simulink model "Dynamic_vibration_absorber"  (R2020b)
settings: Solver=VariableStepAuto  StartTime=0.0  StopTime=10  RelTol=1e-3
PreLoadFcn:
  | %Problem 1 - Dynamic vibration absorber
  | %Values for the model
  | 
  | b=50
  | k1=50
  | k12=50
  | m1=100
  | m2=100
model workspace (MAT data in the model file):
  b = 50
  k1 = 50
  k12 = 50
  m1 = 100
  m2 = 100
settings Model: Creator=user  LastModifiedBy=user

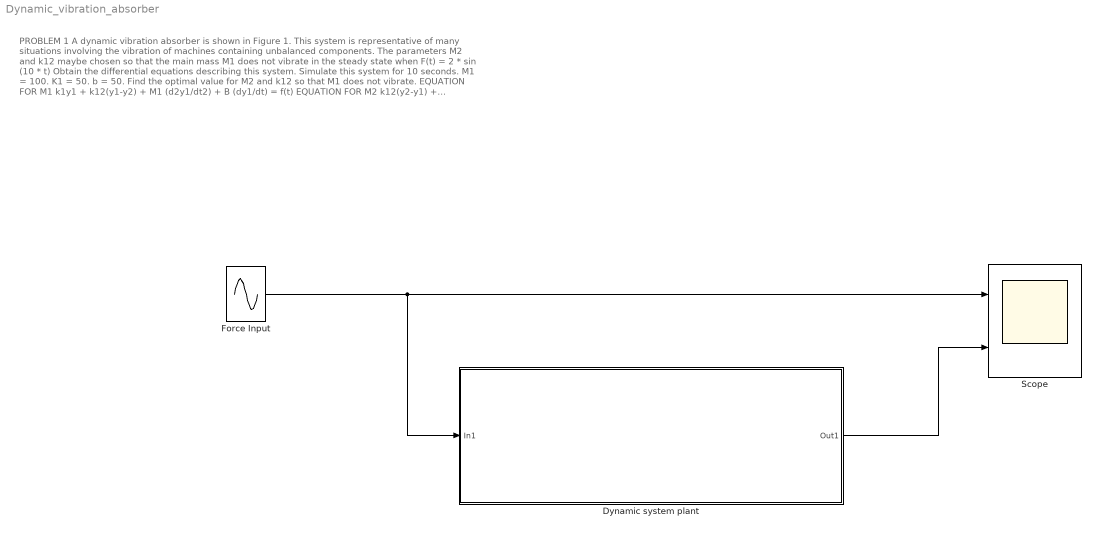
== system Dynamic_vibration_absorber ==
  note: PROBLEM 1
      |
      | A dynamic vibration absorber is shown in Figure 1. This system is representative of many situations involving the vibration of machines containing unbalanced components. The parameters M2 and k12 maybe chosen so that the main mass M1 does not vibrate in the steady state when F(t) = 2 * sin (10 * t) Obtain the differential equations describing this system. Simulate this system for 10 seconds. M1 = 100. K1 = 50. b = 50. Find the optimal value for M2 and k12 so that M1 does not vibrate.
      |
      | EQUATION FOR M1
      | k1y1 + k12(y1-y2) + M1 (d2y1/dt2) + B (dy1/dt) = f(t)
      |
      | EQUATION FOR M2
      | k12(y2-y1) + M2(d2y2/dt2) = 0
  "Dynamic system plant " : Subsystem  mask{m2=4, k12=25}
      mask prompts: m2 "Mass(m2)"; k12 "Spring Constant(k12)"
      mask Display: image('C:\Users\user\Downloads\Screenshot_20210307-220826.jpg'); % Use "Edit Image" on toolstrip to change.
  Force Input : Sin  Amplitude=2  Frequency=10  SampleTime=0
  "Scope " : Scope  NumInputPorts=2
  wires:
  Force Input/1 -> "Dynamic system plant "/1(In1), "Scope "/1
  "Dynamic system plant "/1(Out1) -> "Scope "/2

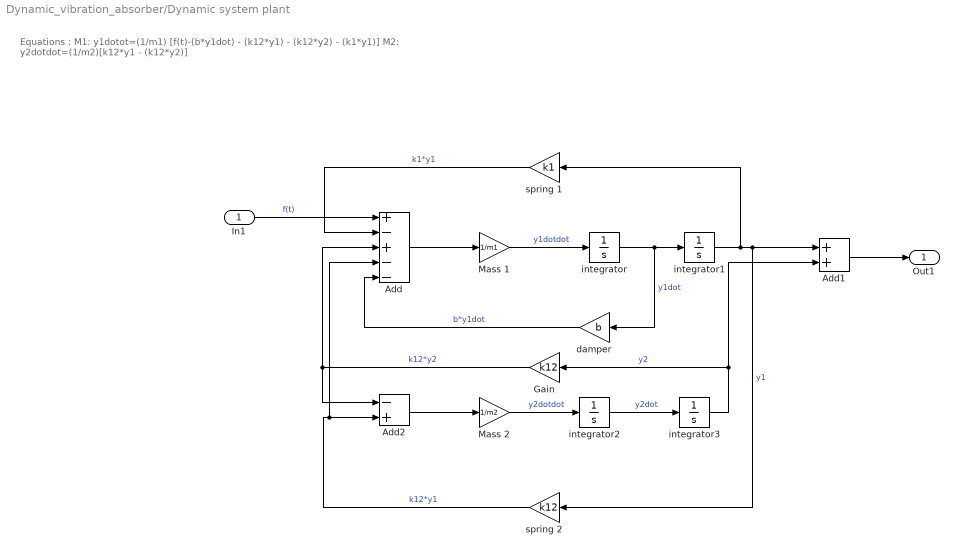
== system Dynamic_vibration_absorber/Dynamic system plant  ==
  note: Equations :
      |
      | M1:
      | y1dotot=(1/m1) [f(t)-(b*y1dot) - (k12*y1) - (k12*y2) - (k1*y1)]
      | M2:
      | y2dotdot=(1/m2)[k12*y1 - (k12*y2)]
  In1 : Inport
  Add : Sum  Inputs=+-+--
  Add1 : Sum
  Add2 : Sum  Inputs=-+
  Gain : Gain  Gain=k12
  Mass 1 : Gain  Gain=1/m1
  Mass 2 : Gain  Gain=1/m2
  damper : Gain  Gain=b
  integrator{,1..3} (4 alike) : Integrator
  spring 1 : Gain  Gain=k1
  spring 2 : Gain  Gain=k12
  Out1 : Outport
  wires:
  Mass 2/1 -> integrator2/1  "y2dotdot"
  integrator/1 -> damper/1, integrator1/1  "y1dot"
  integrator1/1 -> spring 2/1, Add1/1, spring 1/1  "y1"
  Mass 1/1 -> integrator/1  "y1dotdot"
  spring 2/1 -> Add/4, Add2/2  "k12*y1"
  Add/1 -> Mass 1/1
  spring 1/1 -> Add/2  "k1*y1"
  integrator2/1 -> integrator3/1  "y2dot"
  damper/1 -> Add/5  "b*y1dot"
  In1/1 -> Add/1  "f(t)"
  Add1/1 -> Out1/1
  integrator3/1 -> Add1/2, Gain/1  "y2"
  Gain/1 -> Add/3, Add2/1  "k12*y2"
  Add2/1 -> Mass 2/1
